simulink model "rlAOCSModel_one_agent_2022_03_09_reduced_q"  (R2021a)
settings: Solver=FixedStepAuto  StartTime=0.0  StopTime=60  FixedStep=Ts  RelTol=1e-3
values from neighbouring files (symbols this model uses):
  omega_max = 0.015    [AOCS_RL_setup_1_agent_TD3_2022_03_09_reduced_obs.m]
  qe_max = 0.18    [AOCS_RL_setup_1_agent_TD3_2022_03_09_reduced_obs.m]
  qe_min = 0.09    [AOCS_RL_setup_1_agent_TD3_2022_03_09_reduced_obs.m]
libraries: sharedutil x6, dspmtrx3 x1, rllib x1
settings Model: Creator=HP  LastModifiedBy=HP
settings DebuggingCC: AlgebraicLoopMsg=error  ParameterOverflowMsg=none

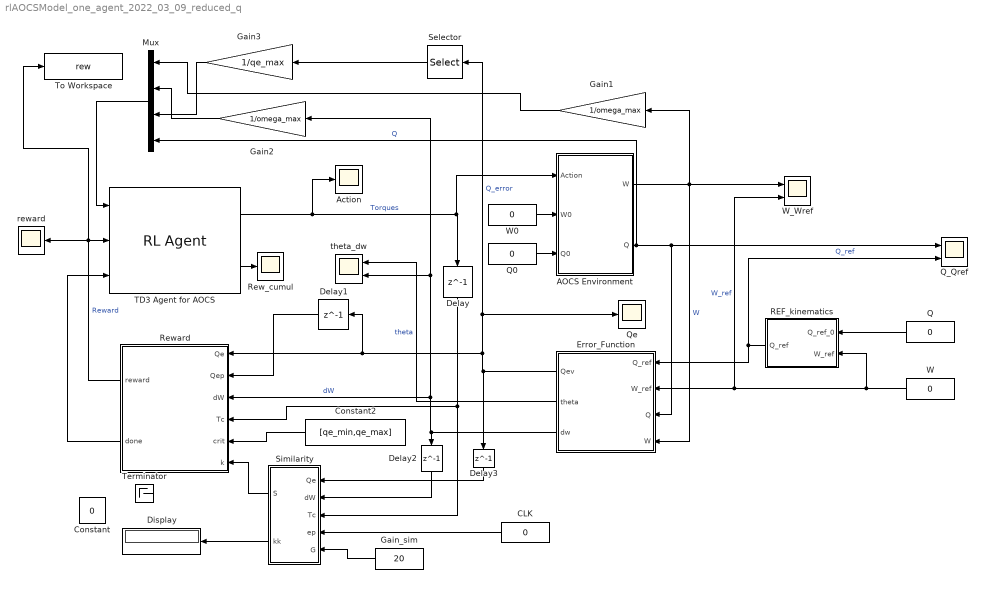
== system rlAOCSModel_one_agent_2022_03_09_reduced_q ==
  AOCS Environment : Subsystem
  Action : Scope
  CLK : Constant  Value=0  SampleTime=Inf
  Constant : Constant  Value=0
  Constant2 : Constant  Value=[qe_min,qe_max]
  Delay{,1..3} (4 alike) : Delay  DelayLength=1
  Display : Display
  Error_Function : MATLAB Function  TreatAsAtomicUnit=on
  Gain1 : Gain  Gain=1/omega_max
  Gain2 : Gain  Gain=1/omega_max
  Gain3 : Gain  Gain=1/qe_max
  Gain_sim : Constant  Value=20  SampleTime=Inf
  Mux : Mux
  Q : Constant  Value=0  SampleTime=Inf
  Q0 : Constant  Value=0  SampleTime=Inf
  Q_Qref : Scope  NumInputPorts=2
  Qe : Scope
  REF_kinematics : Subsystem
  Rew_cumul : Scope
  Reward : MATLAB Function  TreatAsAtomicUnit=on
  Selector : Selector  InputPortWidth=4  IndexOptions=Index vector (dialog)  Indices=[2 3 4]  OutputSizes=3
  Similarity : MATLAB Function  TreatAsAtomicUnit=on
  TD3 Agent for AOCS : rllib/RL Agent  Agent=TD3_AOCS  ExternalActionAsInput=off  ProvideCumRwd=on  TreatAsDirectFeedthrough=on
  Terminator : Terminator
  To Workspace : ToWorkspace  VariableName=rew  SaveFormat=Timeseries  SampleTime=-1
  W : Constant  Value=0  SampleTime=Inf
  W0 : Constant  Value=0  SampleTime=Inf
  W_Wref : Scope  NumInputPorts=2
  reward : Scope
  theta_dw : Scope  NumInputPorts=2
  wires:
  Reward/2(done) -> TD3 Agent for AOCS/3
  Delay/1 -> Reward/4(Tc), Similarity/3(Tc)
  W/1 -> REF_kinematics/2(W_ref), Error_Function/2(W_ref), W_Wref/2  "W_ref"
  Constant2/1 -> Reward/5(crit)
  Reward/1(reward) -> To Workspace/1, reward/1, TD3 Agent for AOCS/2  "Reward"
  Error_Function/3(dw) -> Gain2/1, theta_dw/2, Reward/3(dW), Delay2/1  "dW"
  Error_Function/2(theta) -> theta_dw/1  "theta"
  AOCS Environment/1(W) -> Gain1/1, W_Wref/1, Error_Function/4(W)  "W"
  Error_Function/1(Qev) -> Selector/1, Qe/1, Delay1/1, Reward/1(Qe), Delay3/1  "Q_error"
  AOCS Environment/2(Q) -> Mux/4, Q_Qref/1, Error_Function/3(Q)  "Q"
  REF_kinematics/1(Q_ref) -> Error_Function/1(Q_ref), Q_Qref/2  "Q_ref"
  TD3 Agent for AOCS/2 -> Rew_cumul/1
  Q/1 -> REF_kinematics/1(Q_ref_0)
  Q0/1 -> AOCS Environment/3(Q0)
  CLK/1 -> Similarity/4(ep)
  Gain_sim/1 -> Similarity/5(G)
  Similarity/2(kk) -> Display/1
  Mux/1 -> TD3 Agent for AOCS/1
  Delay1/1 -> Reward/2(Qep)
  Gain1/1 -> Mux/1
  Gain2/1 -> Mux/2
  Selector/1 -> Gain3/1
  TD3 Agent for AOCS/1 -> AOCS Environment/1(Action), Delay/1, Action/1  "Torques"
  W0/1 -> AOCS Environment/2(W0)
  Delay3/1 -> Similarity/1(Qe)
  Delay2/1 -> Similarity/2(dW)
  Gain3/1 -> Mux/3
  Similarity/1(S) -> Reward/6(k)

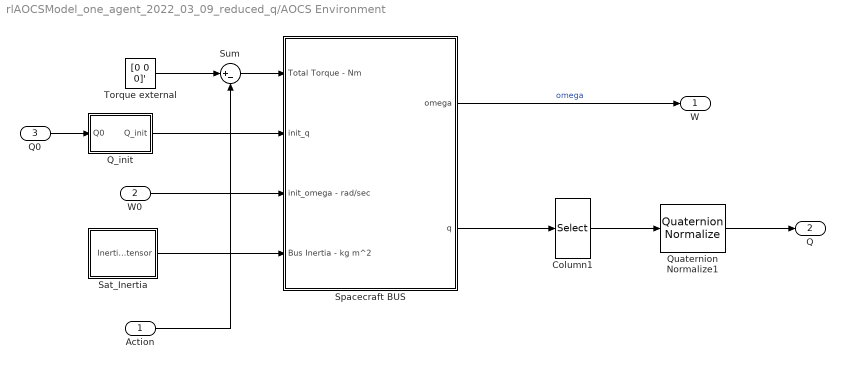
== system rlAOCSModel_one_agent_2022_03_09_reduced_q/AOCS Environment ==
  Action : Inport
  W0 : Inport  Port=2
  Q0 : Inport  Port=3
  Column1 : Selector  InputPortWidth=4  IndexOptions=Index vector (dialog)  Indices=[4 1 2 3]  OutputSizes=1
  Q_init : Subsystem
  Quaternion Normalize1 : sharedutil/Quaternion Normalize  aMode=aMode
      settings: SourceProductBaseCode=AE,PW,DR,MT,UV,VE
  Sat_Inertia : Subsystem
  Spacecraft BUS : Subsystem
  Sum : Sum  Inputs=|+-
  Torque external : Constant  Value=[0 0 0]'
  W : Outport
  Q : Outport  Port=2
  wires:
  Action/1 -> Sum/2
  Sat_Inertia/1(Inertia_tensor) -> Spacecraft BUS/4(Bus Inertia - kg m^2)
  Spacecraft BUS/1(omega) -> W/1  "omega"
  Sum/1 -> Spacecraft BUS/1(Total Torque - Nm)
  W0/1 -> Spacecraft BUS/3(init_omega - rad/sec)
  Torque external/1 -> Sum/1
  Q_init/1(Q_init) -> Spacecraft BUS/2(init_q)
  Spacecraft BUS/2(q) -> Column1/1
  Column1/1 -> Quaternion Normalize1/1
  Quaternion Normalize1/1 -> Q/1
  Q0/1 -> Q_init/1(Q0)

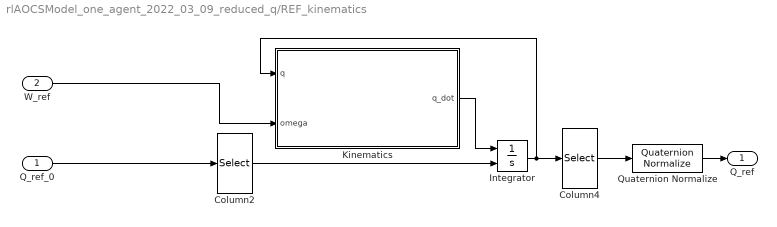
== system rlAOCSModel_one_agent_2022_03_09_reduced_q/REF_kinematics ==
  Q_ref_0 : Inport
  W_ref : Inport  Port=2
  Column2 : Selector  InputPortWidth=4  IndexOptions=Index vector (dialog)  Indices=[2 3 4 1]  OutputSizes=1
  Column4 : Selector  InputPortWidth=4  IndexOptions=Index vector (dialog)  Indices=[4 1 2 3]  OutputSizes=1
  Integrator : Integrator  InitialConditionSource=external
  Kinematics : Subsystem
  Quaternion Normalize : sharedutil/Quaternion Normalize  aMode=aMode
      settings: SourceProductBaseCode=AE,PW,DR,MT,UV,VE
  Q_ref : Outport
  wires:
  Q_ref_0/1 -> Column2/1
  W_ref/1 -> Kinematics/2(omega)
  Column2/1 -> Integrator/2
  Integrator/1 -> Column4/1, Kinematics/1(q)
  Kinematics/1(q_dot) -> Integrator/1
  Column4/1 -> Quaternion Normalize/1
  Quaternion Normalize/1 -> Q_ref/1

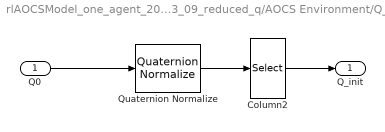
== system rlAOCSModel_one_agent_2022_03_09_reduced_q/AOCS Environment/Q_init ==
  Q0 : Inport
  Column2 : Selector  InputPortWidth=4  IndexOptions=Index vector (dialog)  Indices=[2 3 4 1]  OutputSizes=1
  Quaternion Normalize : sharedutil/Quaternion Normalize  aMode=aMode
      settings: SourceProductBaseCode=AE,PW,DR,MT,UV,VE
  Q_init : Outport
  wires:
  Column2/1 -> Q_init/1
  Q0/1 -> Quaternion Normalize/1
  Quaternion Normalize/1 -> Column2/1

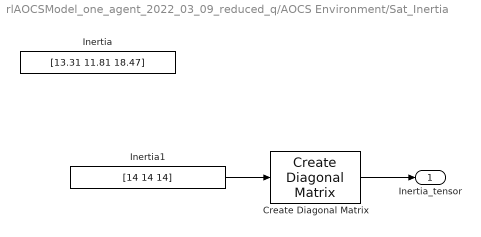
== system rlAOCSModel_one_agent_2022_03_09_reduced_q/AOCS Environment/Sat_Inertia ==
  Create Diagonal Matrix : dspmtrx3/Create Diagonal Matrix
      settings: SourceProductBaseCode=DS
  Inertia : Constant  Value=[13.31 11.81 18.47]
  Inertia1 : Constant  Value=[14 14 14]
  Inertia_tensor : Outport
  wires:
  Create Diagonal Matrix/1 -> Inertia_tensor/1
  Inertia1/1 -> Create Diagonal Matrix/1

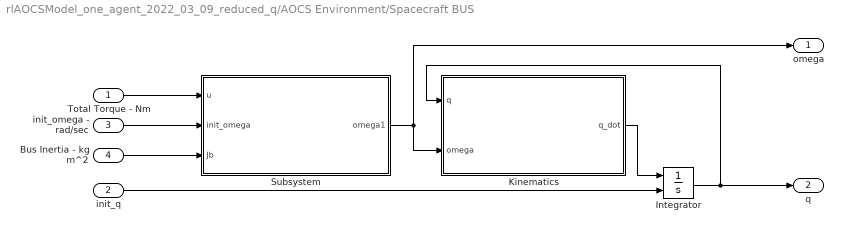
== system rlAOCSModel_one_agent_2022_03_09_reduced_q/AOCS Environment/Spacecraft BUS ==
  Total Torque - Nm : Inport
  init_q : Inport  Port=2
  init_omega - rad/sec : Inport  Port=3
  Bus Inertia - kg m^2 : Inport  Port=4
  Integrator : Integrator  InitialConditionSource=external
  Kinematics : Subsystem
  Subsystem : Subsystem
  omega : Outport  VectorParamsAs1DForOutWhenUnconnected=off
  q : Outport  Port=2  VectorParamsAs1DForOutWhenUnconnected=off
  wires:
  Kinematics/1(q_dot) -> Integrator/1
  Integrator/1 -> Kinematics/1(q), q/1
  Total Torque - Nm/1 -> Subsystem/1(u)
  init_omega - rad/sec/1 -> Subsystem/2(init_omega)
  init_q/1 -> Integrator/2
  Subsystem/1(omega1) -> Kinematics/2(omega), omega/1
  Bus Inertia - kg m^2/1 -> Subsystem/3(Jb)

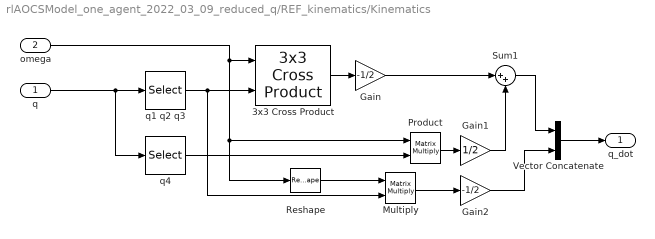
== system rlAOCSModel_one_agent_2022_03_09_reduced_q/REF_kinematics/Kinematics ==
  q : Inport
  omega : Inport  Port=2
  3x3 Cross Product : sharedutil/3x3 Cross Product  aMode=aMode
      settings: SourceProductBaseCode=AE,PW,DR,MT,UV,VE
  Gain : Gain  Gain=-1/2
  Gain1 : Gain  Gain=1/2
  Gain2 : Gain  Gain=-1/2
  Multiply : Product  Multiplication=Matrix(*)
  Product : Product  Multiplication=Matrix(*)
  Reshape : Reshape  OutputDimensionality=Row vector (2-D)
  Sum1 : Sum  Inputs=|++
  Vector Concatenate : Concatenate
  q1 q2 q3 : Selector  InputPortWidth=4  IndexOptions=Index vector (dialog)  Indices=[1 2 3]  OutputSizes=1
  q4 : Selector  InputPortWidth=4  IndexOptions=Index vector (dialog)  Indices=[4]  OutputSizes=1
  q_dot : Outport  VectorParamsAs1DForOutWhenUnconnected=off
  wires:
  omega/1 -> 3x3 Cross Product/1, Product/1, Reshape/1
  q/1 -> q4/1, q1 q2 q3/1
  q1 q2 q3/1 -> Multiply/2, 3x3 Cross Product/2
  Gain1/1 -> Sum1/2
  3x3 Cross Product/1 -> Gain/1
  Product/1 -> Gain1/1
  Multiply/1 -> Gain2/1
  Gain/1 -> Sum1/1
  q4/1 -> Product/2
  Sum1/1 -> Vector Concatenate/1
  Gain2/1 -> Vector Concatenate/2
  Reshape/1 -> Multiply/1
  Vector Concatenate/1 -> q_dot/1

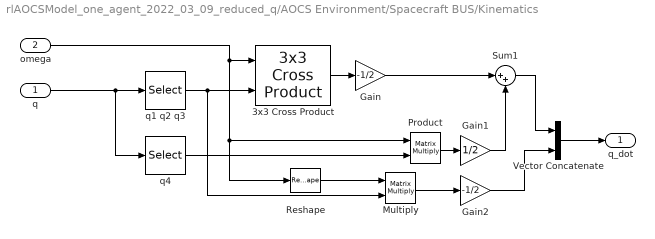
== system rlAOCSModel_one_agent_2022_03_09_reduced_q/AOCS Environment/Spacecraft BUS/Kinematics ==
  q : Inport
  omega : Inport  Port=2
  3x3 Cross Product : sharedutil/3x3 Cross Product  aMode=aMode
      settings: SourceProductBaseCode=AE,PW,DR,MT,UV,VE
  Gain : Gain  Gain=-1/2
  Gain1 : Gain  Gain=1/2
  Gain2 : Gain  Gain=-1/2
  Multiply : Product  Multiplication=Matrix(*)
  Product : Product  Multiplication=Matrix(*)
  Reshape : Reshape  OutputDimensionality=Row vector (2-D)
  Sum1 : Sum  Inputs=|++
  Vector Concatenate : Concatenate
  q1 q2 q3 : Selector  InputPortWidth=4  IndexOptions=Index vector (dialog)  Indices=[1 2 3]  OutputSizes=1
  q4 : Selector  InputPortWidth=4  IndexOptions=Index vector (dialog)  Indices=[4]  OutputSizes=1
  q_dot : Outport  VectorParamsAs1DForOutWhenUnconnected=off
  wires:
  omega/1 -> 3x3 Cross Product/1, Product/1, Reshape/1
  q/1 -> q4/1, q1 q2 q3/1
  q1 q2 q3/1 -> Multiply/2, 3x3 Cross Product/2
  Gain1/1 -> Sum1/2
  3x3 Cross Product/1 -> Gain/1
  Product/1 -> Gain1/1
  Multiply/1 -> Gain2/1
  Gain/1 -> Sum1/1
  q4/1 -> Product/2
  Sum1/1 -> Vector Concatenate/1
  Gain2/1 -> Vector Concatenate/2
  Reshape/1 -> Multiply/1
  Vector Concatenate/1 -> q_dot/1

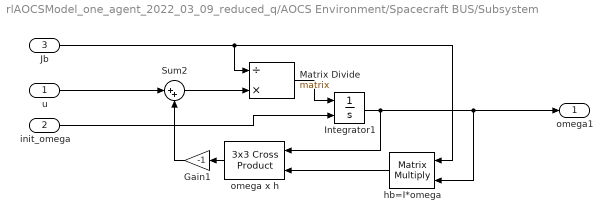
== system rlAOCSModel_one_agent_2022_03_09_reduced_q/AOCS Environment/Spacecraft BUS/Subsystem ==
  u : Inport
  init_omega : Inport  Port=2
  Jb : Inport  Port=3
  Gain1 : Gain  Gain=-1
  Integrator1 : Integrator  InitialConditionSource=external  ZeroCross=off
  Matrix Divide : Product  Inputs=/*  Multiplication=Matrix(*)
  Sum2 : Sum  Inputs=|++
  hb=I*omega : Product  Multiplication=Matrix(*)
  omega x h : sharedutil/3x3 Cross Product  aMode=aMode
      settings: SourceProductBaseCode=AE,PW,DR,MT,UV,VE
  omega1 : Outport  VectorParamsAs1DForOutWhenUnconnected=off
  wires:
  Gain1/1 -> Sum2/2
  Integrator1/1 -> omega x h/1, omega1/1, hb=I*omega/2
  init_omega/1 -> Integrator1/2
  Sum2/1 -> Matrix Divide/2
  hb=I*omega/1 -> omega x h/2
  omega x h/1 -> Gain1/1
  u/1 -> Sum2/1
  Matrix Divide/1 -> Integrator1/1
  Jb/1 -> Matrix Divide/1, hb=I*omega/1

== matlab function rlAOCSModel_one_agent_2022_03_09_reduced_q/Similarity ==
  data: S output size=1; Qe input; dW input; Tc input; ep input; G input; kk output size=1
function [S,kk] = Similarity(Qe,dW,Tc,ep,G)
%[S,PTc,Dist,crs]
% Inputs:
% Qe(1x4 real array): Quaternion of error
% dW(1x3 real array): Omega error
% Tc(1x3 real array): Last applied torque
% ep(integer): Episode number after which no more similarity measure.
%       ==> After this value, the standard reward is used.
% distrib(string): Statistical distribution used to evaluate similarity.
%       Values: 'Gauss', 'Burr', 'None'.
% G: gain. In principle, max output similarity measure is 1.
%       ==> This param is used to scale the max output.
distrib = 'Gauss';%'None';%'Burr';%
kk = 0;
if ep < 500
% Parameters definition
% PD Gains
    Kp = .6;%
    Kd = 3.6;%
    Tlim = 0.012; % torques limit
    S_th = 5e-5; % thershold of similarity
% Gaussian function
    sigma = S_th/1; % std (sigma is minimized to rise high value detectability near zero.)
    mean = 0;% mean
% Burr distribution
    alpha = S_th/5;
    c = 10;
    k = .5;
% Compute PD torque
    PTc = (Qe(2:4) * Kp) + (dW * Kd);
% saturation of torques
    PTc = min(PTc,Tlim*ones(size(PTc)));
    PTc = max(PTc,-Tlim*ones(size(PTc)));
% Compute euclidean distances w.r.t Agent torques
% Dist = sqrt(sum((PTc-Tc).^2));
% Use the cross product as inverse similarity metric
% When minimal, the vectors are more close. 
    crsV = cross(PTc,Tc);
% validity to use the cross product only when at most
% one coordinate has the sign changed.
    if sum(sign(PTc.*Tc)) == 3
        crs = norm(crsV);
    else
        crs = 1; % high value to the right to decrease output value.
    end

    if strcmp(distrib, 'Gauss')
        S = G*gaussian(crs,sigma,mean);
        kk = 2;
    end

    if strcmp(distrib, 'Burr')
        S = G*inv_burr_cdf(crs,alpha,c,k);
        kk = 1;
    end
    
    if strcmp(distrib, 'None')
        S = G;
    end

else % Remaining Episodes of training, no more reward adjustment.
    S = 0;
end

function g = gaussian(value,sigma,mean)
%weighted gaussian function 
    g = exp(-.5*(((value-mean)/sigma)^2));
end

function g = inv_burr_cdf(value,alpha,c,k)
%inverted burr cdf ==> 1 - burr_cdf. 
%     g = 1 - cdf('burr',value,alpha,c,k);
    g = (1+(value/alpha).^c).^-k;
end

end

== matlab function rlAOCSModel_one_agent_2022_03_09_reduced_q/Error_Function ==
  data: Qev output; Q_ref input; theta output; W_ref input; dw output; Q input; W input
function [Qev, theta, dw]= error(Q_ref,W_ref,Q, W)
% Compute angle/velocity errors
Qt = Q';
Q1 = quatconj(Q_ref');
Q2 = quatmultiply(Q1,Qt);
Qe = quatnormalize(Q2);
Q1 = quatmultiply([0,W_ref'],Qe);
Q2 = quatconj(Qe);
Q3 = quatmultiply(Q2,Q1);
Wr = Q3(2:4);
% dW computed like ALSAT (with Quat involved)
dw = W - Wr';
% dW computed as difference
% dw = W_ref' - W; 
s = 2 * sign(Qe(1));
theta = s * Qe(2:4);
Qev = Qe';

== matlab function rlAOCSModel_one_agent_2022_03_09_reduced_q/Reward ==
  data: Qe input; Qep input; dW input; Tc input; crit input; reward output; done output; k input
function [reward,done] = Reward(Qe,Qep,dW,Tc,crit,k)
d = false;

tnorm = 2;
Qv = Qe(2:4);
% Qvp = Qep(2:4);
% sigma = 2e-3;
% reward = exp(-.5*(((norm(Qv,tnorm))/sigma)^2));
reward = -norm(Qv,tnorm)-norm(Tc,tnorm);%-norm(dW,tnorm);
if norm(Qv,Inf) <= crit(1)
    reward = reward + (1/(0.01+(norm(Qv,tnorm))));
%     reward = reward + exp(-.5*(((norm(dW,tnorm))/sigma)^2));
end

reward = reward + k ;
if norm(Qv,Inf) >  crit(2)
    reward = -150;
    d = true;
end

done = d;
end


% function g = w_g(gain,value,sigma)
% %weighted gaussian function 
% g = gain*exp(-.5*((value/sigma)^2))/(sigma*sqrt(2*pi));
% end
